simulink model "Copy_of_LQR_bloques_SS_LQR_cascada_PID_controller"  (R2023a)
settings: Solver=VariableStepAuto  StartTime=0.0  StopTime=2000  RelTol=1e-3
undefined symbols (not defined in the file): A, A_model, A_motor, B, B_mag0, B_model2, B_motor, C_model2, C_motor, D_motor, Gamma, I, J, K3_2, K4_2, K_gamma, Ke, Kt, La, n_cal, R_mgt, Ra, T_ext, T_max, T_max_mgt
libraries: slpidlib x7, matrix_library x5, simulink_extras x3, aerolibutil x1, vrlib x1
settings Model: Creator=Personal  LastModifiedBy=Personal
settings SolverCC: ZeroCrossAlgorithm=Adaptive
settings DebuggingCC: MaskedZcDiagnostic=none  IgnoredZcDiagnostic=none

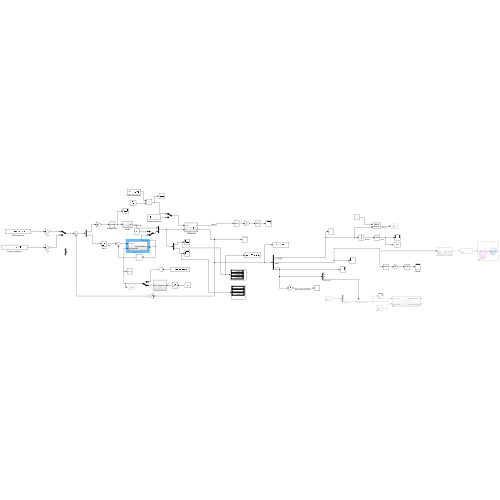
[thumbnail: Simulink's stored preview of the top-level diagram]
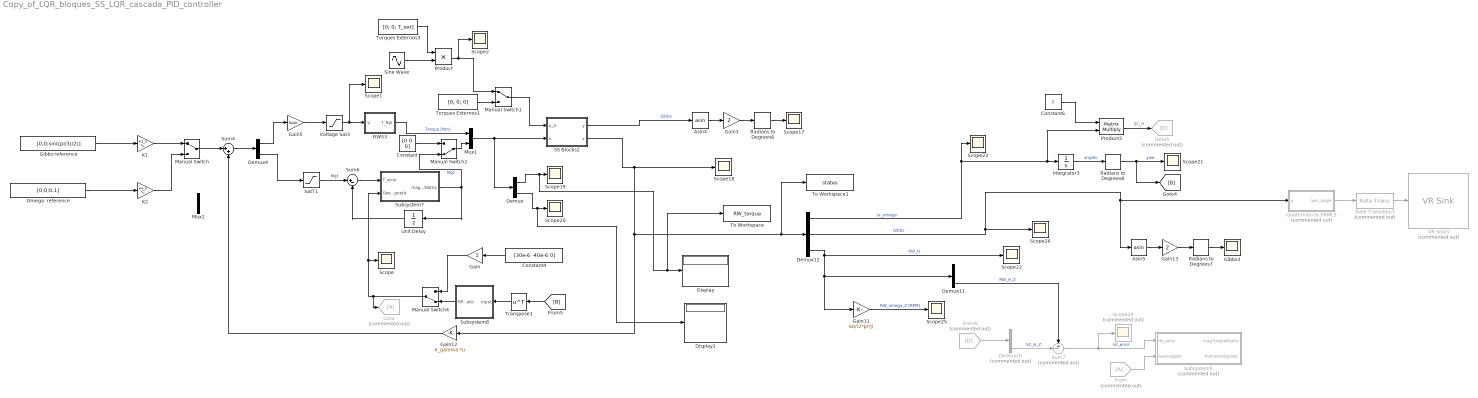
== system Copy_of_LQR_bloques_SS_LQR_cascada_PID_controller ==
  Asin4 : Trigonometry  Operator=asin
  Asin5 : Trigonometry  Operator=asin
  Constant : Constant  Value=[0 0 0]
  Constant4 : Constant  Value=[30e-6 -40e-6 0]
  Constant6 : Constant  Value=I
  Demux : Demux  Outputs=2
  Demux10 : Demux  Commented=on  Outputs=3
  Demux11 : Demux  Outputs=3
  Demux12 : Demux  Outputs=3
  Demux4 : Demux  Outputs=2
  Display : Display
  Display1 : Display
  From : From  Commented=on
  From6 : From  Commented=on  GotoTag=D
  Gain : Gain
  Gain11 : Gain  Gain=60/(2*pi*J)
  Gain12 : Gain  Gain=-K_gamma  Multiplication=Matrix(K*u)
  Gain13 : Gain  Gain=2
  Gain3 : Gain  Gain=2
  Gain5 : Gain  Gain=Ra/Kt
  Gibbs reference : Constant  Value=[0;0;sin((pi/3)/2)]
  Gibbs3 : Scope
  Goto : Goto  Commented=on
  Goto5 : Goto  Commented=on  GotoTag=D
  Integrator3 : Integrator  InitialCondition=[0 0 0]
  K1 : Gain  Gain=K3_2  Multiplication=Matrix(K*u)
  K2 : Gain  Gain=K4_2  Multiplication=Matrix(K*u)
  Manual Switch : ManualSwitch
  Manual Switch1 : ManualSwitch
  Manual Switch2 : ManualSwitch  CurrentSetting=0
  Manual Switch4 : ManualSwitch  CurrentSetting=0
  Mux1 : Mux  Inputs=2
  Mux2 : Mux  Inputs=2
  Omega  reference : Constant  Value=[0;0;0.1]
  Product : Product
  Product3 : Product  Multiplication=Matrix(*)
  Quaternion to VRML3 : Subsystem  Commented=on
  RWS3 : Subsystem
  Radians to Degrees6 : simulink_extras/Transformations/Radians to Degrees
  Radians to Degrees7 : simulink_extras/Transformations/Radians to Degrees
  Radians to Degrees8 : simulink_extras/Transformations/Radians to Degrees
  Rate Transition3 : RateTransition  Commented=on
  SS Blocks2 : Subsystem
  SatT1 : Saturate  UpperLimit=T_max_mgt  LowerLimit=-T_max_mgt
  Scope{,1..2,17..23,25..26} (12 alike) : Scope
  Scope24 : Scope  Commented=on
  Sine Wave : Sin  Frequency=0.05  SampleTime=0
  Subsystem7 : Subsystem
  Subsystem8 : Subsystem
  Subsystem9 : Subsystem  Commented=on
  Sum4 : Sum  Inputs=|++
  Sum6 : Sum  Inputs=|+-
  Sum7 : Sum  Commented=on  Inputs=+-|
  To Workspace : ToWorkspace  VariableName=RW_torque  SaveFormat=Structure With Time  SampleTime=-1
  To Workspace1 : ToWorkspace  VariableName=states  SaveFormat=Structure With Time  SampleTime=-1
  Torques Externos1 : Constant  Value=[0; 0; 0]
  Torques Externos3 : Constant  Value=[0; 0; T_ext]
  Transpose1 : Math  Operator=transpose
  Unit Delay : UnitDelay  SampleTime=-1  HasFrameUpgradeWarning=on
  VR Sink3 : vrlib/VR Sink  Commented=on  InstantiateOnLoad=on  SampleTime=0.1  ViewEnable=on  RemoteChange=off  RemoteView=off  FieldsWritten=STLB_Transform.rotation.4.1.1.double  WorldFileName=EscenarioCubeSat.x3d  AutoView=off  VideoDimensions=[]  AllowVariableSize=off  FigureProperties=[]
  Voltage Sat3 : Saturate  UpperLimit=6  LowerLimit=-6
  wires:
  Gibbs reference/1 -> K1/1
  K1/1 -> Manual Switch/1
  Mux1/1 -> Demux/1, SS Blocks2/2(u)
  Torques Externos3/1 -> Product/1
  Gain3/1 -> Radians to Degrees6/1
  SS Blocks2/1(y) -> Asin4/1  "Gibbs"
  Asin4/1 -> Gain3/1
  Radians to Degrees6/1 -> Scope17/1
  Demux/1 -> To Workspace/1, Display/1, Scope19/1
  Demux/2 -> Display1/1, Scope20/1
  Voltage Sat3/1 -> Scope1/1, RWS3/1(V)
  Gain5/1 -> Voltage Sat3/1
  SatT1/1 -> Sum6/1  "Mgt"
  Sum6/1 -> Subsystem7/1(T_error)
  Manual Switch4/1 -> Goto/1, Scope/1, Subsystem7/2(Geomagnetic)
  Demux4/1 -> Gain5/1
  Demux4/2 -> SatT1/1
  Gain12/1 -> Sum4/2
  Sum4/1 -> Demux4/1
  Subsystem7/1(magTorqueMatrix) -> Manual Switch2/2, Unit Delay/1  "Mgt"
  RWS3/1(T_RW) -> Mux1/1  "Torque [Nm]"
  Constant4/1 -> Gain/1
  Subsystem8/1(RPY_Magnetic) -> Manual Switch4/2
  Transpose1/1 -> Subsystem8/1(Input)
  Gain/1 -> Manual Switch4/1
  From6/1 -> Demux10/1
  SS Blocks2/2(x) -> Gain12/1, To Workspace1/1, Demux12/1, Scope18/1
  Radians to Degrees7/1 -> Gibbs3/1
  Demux10/3 -> Sum7/2  "SC_H_Z"
  Radians to Degrees8/1 -> [B], Scope21/1  "yaw"
  Demux11/3 -> Sum7/1  "RW_H_Z"
  Rate Transition3/1 -> VR Sink3/1
  Quaternion to VRML3/1(axis_angle) -> Rate Transition3/1
  Gain13/1 -> Radians to Degrees7/1
  Product3/1 -> Goto5/1  "SC_H"
  Integrator3/1 -> Radians to Degrees8/1  "angles"
  Gain11/1 -> Scope25/1  "RW_omega_Z [RPM]"
  Demux12/2 -> Asin5/1, Quaternion to VRML3/1(q), Scope26/1  "Gibbs"
  Sum7/1 -> Scope24/1, Subsystem9/1(Hz_error)  "Hz_error"
  Asin5/1 -> Gain13/1
  Constant6/1 -> Product3/1
  Demux12/3 -> Scope22/1, Gain11/1, Demux11/1  "RW_H"
  Demux12/1 -> Integrator3/1, Product3/2, Scope23/1  "sc_omega"
  [B] -> Transpose1/1
  Unit Delay/1 -> Sum6/2
  From/1 -> Subsystem9/2(Geomagetic)
  Omega  reference/1 -> K2/1
  Manual Switch/1 -> Sum4/1
  K2/1 -> Manual Switch/2
  Manual Switch1/1 -> SS Blocks2/1(u_d)
  Torques Externos1/1 -> Manual Switch1/2
  Constant/1 -> Manual Switch2/1
  Manual Switch2/1 -> Mux1/2
  Sine Wave/1 -> Product/2
  Product/1 -> Scope2/1, Manual Switch1/1

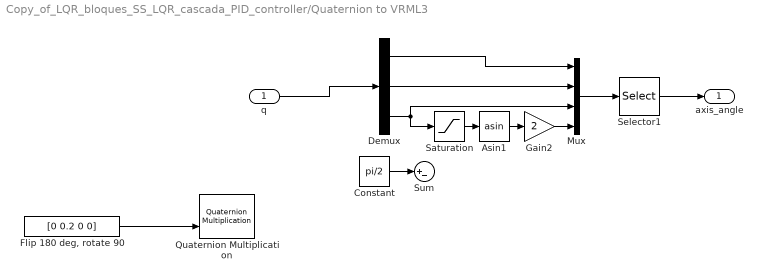
== system Copy_of_LQR_bloques_SS_LQR_cascada_PID_controller/Quaternion to VRML3 ==
  q : Inport
  Asin1 : Trigonometry  Operator=asin
  Constant : Constant  Value=pi/2
  Demux : Demux  Outputs=3
  "Flip 180 deg, rotate 90" : Constant  Value=[0 0.2 0 0]
  Gain2 : Gain  Gain=2
  Mux : Mux
  Quaternion Multiplication : aerolibutil/Quaternion Multiplication
  Saturation : Saturate
  Selector1 : Selector  InputPortWidth=4  IndexOptions=Index vector (dialog)  Indices=[2 3 1 4]  OutputSizes=1
  Sum : Sum  Inputs=|+-
  axis_angle : Outport  VectorParamsAs1DForOutWhenUnconnected=off
  wires:
  Constant/1 -> Sum/1
  Saturation/1 -> Asin1/1
  Asin1/1 -> Gain2/1
  Demux/3 -> Mux/3, Saturation/1
  Gain2/1 -> Mux/4
  Selector1/1 -> axis_angle/1
  Mux/1 -> Selector1/1
  Demux/1 -> Mux/1
  q/1 -> Demux/1
  "Flip 180 deg, rotate 90"/1 -> Quaternion Multiplication/2
  Demux/2 -> Mux/2

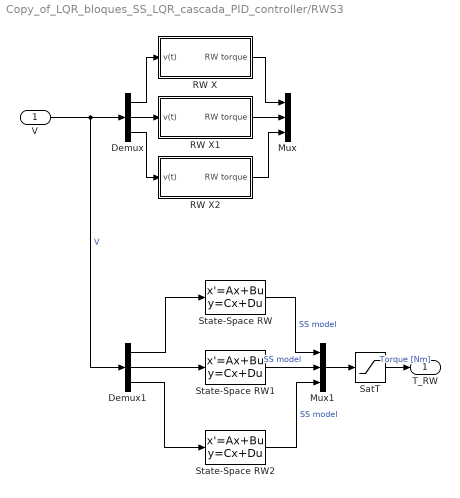
== system Copy_of_LQR_bloques_SS_LQR_cascada_PID_controller/RWS3 ==
  V : Inport
  Demux : Demux  Outputs=3
  Demux1 : Demux  Outputs=3
  Mux : Mux  Inputs=3
  Mux1 : Mux  Inputs=3
  RW X : Subsystem
  RW X1 : Subsystem
  RW X2 : Subsystem
  SatT : Saturate  UpperLimit=T_max  LowerLimit=-T_max
  State-Space RW : StateSpace  A=A_motor  B=B_motor  C=C_motor  D=D_motor  InitialCondition=0
  State-Space RW1 : StateSpace  A=A_motor  B=B_motor  C=C_motor  D=D_motor  InitialCondition=0
  State-Space RW2 : StateSpace  A=A_motor  B=B_motor  C=C_motor  D=D_motor  InitialCondition=0
  T_RW : Outport
  wires:
  Demux/1 -> RW X/1(v(t))
  V/1 -> Demux1/1, Demux/1  "V"
  Demux/3 -> RW X2/1(v(t))
  Demux/2 -> RW X1/1(v(t))
  RW X1/1(RW torque) -> Mux/2
  RW X2/1(RW torque) -> Mux/3
  RW X/1(RW torque) -> Mux/1
  Demux1/1 -> State-Space RW/1
  Demux1/2 -> State-Space RW1/1
  Demux1/3 -> State-Space RW2/1
  State-Space RW1/1 -> Mux1/2  "SS model"
  State-Space RW/1 -> Mux1/1  "SS model"
  State-Space RW2/1 -> Mux1/3  "SS model"
  Mux1/1 -> SatT/1
  SatT/1 -> T_RW/1  "Torque [Nm]"

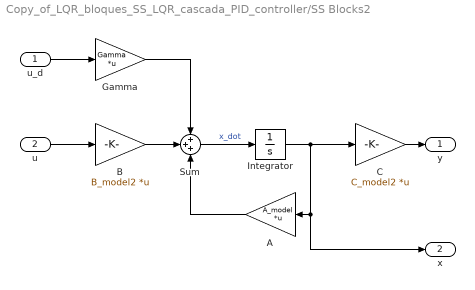
== system Copy_of_LQR_bloques_SS_LQR_cascada_PID_controller/SS Blocks2 ==
  u_d : Inport
  u : Inport  Port=2
  A : Gain  Gain=A_model  Multiplication=Matrix(K*u)
  B : Gain  Gain=B_model2  Multiplication=Matrix(K*u)
  C : Gain  Gain=C_model2  Multiplication=Matrix(K*u)
  Gamma : Gain  Gain=Gamma  Multiplication=Matrix(K*u)
  Integrator : Integrator  InitialCondition=zeros(9,1)
  Sum : Sum  Inputs=+++
  y : Outport
  x : Outport  Port=2
  wires:
  B/1 -> Sum/2
  u/1 -> B/1
  Sum/1 -> Integrator/1  "x_dot"
  A/1 -> Sum/3
  C/1 -> y/1
  Integrator/1 -> C/1, x/1, A/1
  u_d/1 -> Gamma/1
  Gamma/1 -> Sum/1

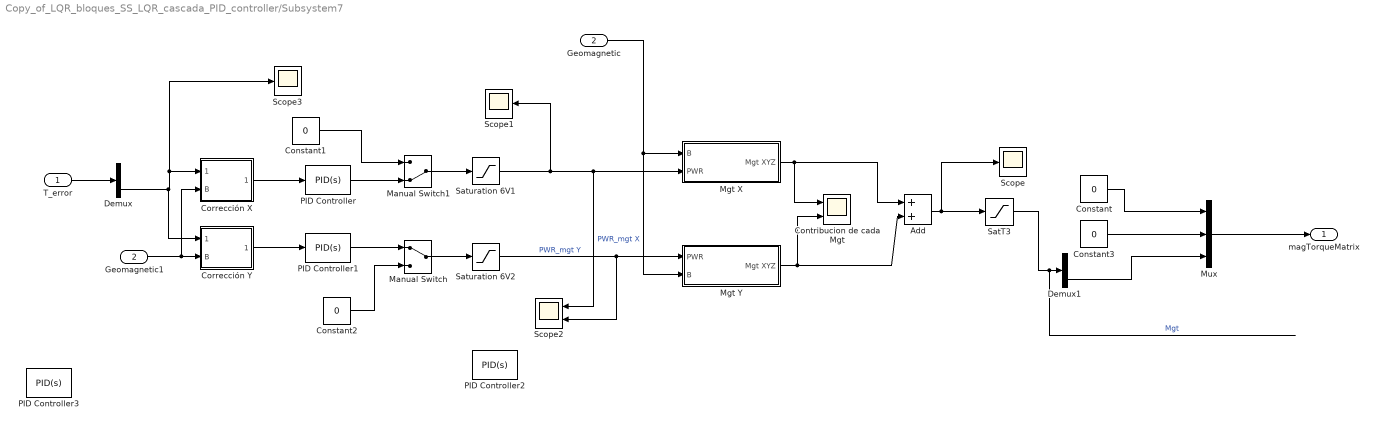
== system Copy_of_LQR_bloques_SS_LQR_cascada_PID_controller/Subsystem7 ==
  T_error : Inport
  Geomagnetic : Inport  Port=2
  Add : Sum
  Constant{,1..3} (4 alike) : Constant  Value=0
  Contribucion de cada Mgt : Scope  NumInputPorts=2
  Corrección X : MATLAB Function  TreatAsAtomicUnit=on
  Corrección Y : MATLAB Function  TreatAsAtomicUnit=on
  Demux : Demux  Outputs=3
  Demux1 : Demux  Outputs=3
  Geomagnetic1 : InportShadow  Port=2
  Manual Switch : ManualSwitch
  Manual Switch1 : ManualSwitch  CurrentSetting=0
  Mgt X : Subsystem
  Mgt Y : Subsystem
  Mux : Mux  Inputs=3
  PID Controller : slpidlib/PID Controller  Controller=PID  Form=Parallel  TimeDomain=Continuous-time  UseExternalTs=off  SampleTime=-1  IntegratorMethod=Forward Euler  FilterMethod=Forward Euler  ControllerParametersSource=internal  P=45000  I=500000  UseKiTs=off  D=8000  N=100  UseFilter=on  TunerSelectOption=Transfer Function Based (PID Tuner App)  InitialConditionSource=internal  InitialConditionForIntegrator=0  InitialConditionForFilter=0  DifferentiatorICPrevScaledInput=0  ExternalReset=none  TrackingMode=off  Kt=1  LimitOutput=on  SatLimitsSource=internal  UpperSaturationLimit=5  LowerSaturationLimit=-5  LinearizeAsGain=on  AntiWindupMode=none  Kb=1  LimitIntegrator=off  UpperIntegratorSaturationLimit=inf  LowerIntegratorSaturationLimit=-inf  POutMin=[]  POutMax=[]  IOutMin=[]  IOutMax=[]  DOutMin=[]  DOutMax=[]  NOutMin=[]  NOutMax=[]  SumOutMin=[]  SumOutMax=[]  SaturationOutMin=[]  SaturationOutMax=[]  PParamMin=[]  PParamMax=[]  IParamMin=[]  IParamMax=[]  DParamMin=[]  DParamMax=[]  NParamMin=[]  NParamMax=[]  KbParamMin=[]  KbParamMax=[]  KtParamMin=[]  KtParamMax=[]  KbOutMin=[]  KbOutMax=[]  KtOutMin=[]  KtOutMax=[]  IntegratorOutMin=[]  IntegratorOutMax=[]  FilterOutMin=[]  FilterOutMax=[]  SumI1OutMin=[]  SumI1OutMax=[]  SumI2OutMin=[]  SumI2OutMax=[]  SumI3OutMin=[]  SumI3OutMax=[]  SumI4OutMin=[]  SumI4OutMax=[]  SumDOutMin=[]  SumDOutMax=[]  DifferentiatorOutMin=[]  DifferentiatorOutMax=[]  FilterDiffOutCoefMin=[]  FilterDiffOutCoefMax=[]  ReciprocalOutMin=[]  ReciprocalOutMax=[]  SumDenOutMin=[]  SumDenOutMax=[]  SumNumOutMin=[]  SumNumOutMax=[]  DivideOutMin=[]  DivideOutMax=[]  UdiffTsProdOutMin=[]  UdiffTsProdOutMax=[]  NTsProdOutMin=[]  NTsProdOutMax=[]  UintegralTsProdOutMin=[]  UintegralTsProdOutMax=[]  UngainTsProdOutMin=[]  UngainTsProdOutMax=[]  ClampingZeroOutDataTypeStr=Inherit: Inherit via back propagation  ClampingZeroOutMin=[]  ClampingZeroOutMax=[]  FilterDenConstantOutDataTypeStr=Inherit: Inherit via back propagation  FilterDenConstantOutMin=[]  FilterDenConstantOutMax=[]  PCopyOutDataTypeStr=Inherit: Inherit via back propagation  PCopyOutMin=[]  PCopyOutMax=[]  NCopyOutDataTypeStr=Inherit: Inherit via back propagation  NCopyOutMin=[]  NCopyOutMax=[]  IntegratorContinuousStateAttributes=''  IntegratorStateMustResolveToSignalObject=off  IntegratorRTWStateStorageClass=Auto  FilterContinuousStateAttributes=''  FilterStateMustResolveToSignalObject=off  FilterRTWStateStorageClass=Auto  ParallelPVariant=InternalParameters  IdealPVariant=Disabled  IVariant=InternalParameters  DVariant=InternalParameters  IntegratorVariant=Continuous  SatVariant=Enabled  AWVariant=Passthrough  PCopyVariant=Disabled  TRVariant=Disabled  FdbkBlocksVariant=Forward  IdealPFdbkVariant=Disabled  SatFdbkVariant=Disabled  DerivativeFilterVariant=ContFilter  NVariant=InternalParameters  NCopyVariant=Disabled  FilterICVariant=InternalICsFilter  IntegratorICVariant=InternalICs  ExternalResetVariant=Disabled  TRSumVariant=Passthrough  SumFdbkVariant=Disabled  SumVariant=Sum_PID  TsampFilterVariant=InternalTs  TsampNgainVariant=Passthrough  TsampIntegralVariant=Disabled_SignalSpec  ExternalSaturationOutDataTypeStr=Inherit: Same as second input
  PID Controller1 : slpidlib/PID Controller  Controller=PID  Form=Parallel  TimeDomain=Continuous-time  UseExternalTs=off  SampleTime=-1  IntegratorMethod=Forward Euler  FilterMethod=Forward Euler  ControllerParametersSource=internal  P=45000  I=500000  UseKiTs=off  D=8000  N=100  UseFilter=on  TunerSelectOption=Transfer Function Based (PID Tuner App)  InitialConditionSource=internal  InitialConditionForIntegrator=0  InitialConditionForFilter=0  DifferentiatorICPrevScaledInput=0  ExternalReset=none  TrackingMode=off  Kt=1  LimitOutput=on  SatLimitsSource=internal  UpperSaturationLimit=5  LowerSaturationLimit=-5  LinearizeAsGain=on  AntiWindupMode=none  Kb=1  LimitIntegrator=off  UpperIntegratorSaturationLimit=inf  LowerIntegratorSaturationLimit=-inf  POutMin=[]  POutMax=[]  IOutMin=[]  IOutMax=[]  DOutMin=[]  DOutMax=[]  NOutMin=[]  NOutMax=[]  SumOutMin=[]  SumOutMax=[]  SaturationOutMin=[]  SaturationOutMax=[]  PParamMin=[]  PParamMax=[]  IParamMin=[]  IParamMax=[]  DParamMin=[]  DParamMax=[]  NParamMin=[]  NParamMax=[]  KbParamMin=[]  KbParamMax=[]  KtParamMin=[]  KtParamMax=[]  KbOutMin=[]  KbOutMax=[]  KtOutMin=[]  KtOutMax=[]  IntegratorOutMin=[]  IntegratorOutMax=[]  FilterOutMin=[]  FilterOutMax=[]  SumI1OutMin=[]  SumI1OutMax=[]  SumI2OutMin=[]  SumI2OutMax=[]  SumI3OutMin=[]  SumI3OutMax=[]  SumI4OutMin=[]  SumI4OutMax=[]  SumDOutMin=[]  SumDOutMax=[]  DifferentiatorOutMin=[]  DifferentiatorOutMax=[]  FilterDiffOutCoefMin=[]  FilterDiffOutCoefMax=[]  ReciprocalOutMin=[]  ReciprocalOutMax=[]  SumDenOutMin=[]  SumDenOutMax=[]  SumNumOutMin=[]  SumNumOutMax=[]  DivideOutMin=[]  DivideOutMax=[]  UdiffTsProdOutMin=[]  UdiffTsProdOutMax=[]  NTsProdOutMin=[]  NTsProdOutMax=[]  UintegralTsProdOutMin=[]  UintegralTsProdOutMax=[]  UngainTsProdOutMin=[]  UngainTsProdOutMax=[]  ClampingZeroOutDataTypeStr=Inherit: Inherit via back propagation  ClampingZeroOutMin=[]  ClampingZeroOutMax=[]  FilterDenConstantOutDataTypeStr=Inherit: Inherit via back propagation  FilterDenConstantOutMin=[]  FilterDenConstantOutMax=[]  PCopyOutDataTypeStr=Inherit: Inherit via back propagation  PCopyOutMin=[]  PCopyOutMax=[]  NCopyOutDataTypeStr=Inherit: Inherit via back propagation  NCopyOutMin=[]  NCopyOutMax=[]  IntegratorContinuousStateAttributes=''  IntegratorStateMustResolveToSignalObject=off  IntegratorRTWStateStorageClass=Auto  FilterContinuousStateAttributes=''  FilterStateMustResolveToSignalObject=off  FilterRTWStateStorageClass=Auto  ParallelPVariant=InternalParameters  IdealPVariant=Disabled  IVariant=InternalParameters  DVariant=InternalParameters  IntegratorVariant=Continuous  SatVariant=Enabled  AWVariant=Passthrough  PCopyVariant=Disabled  TRVariant=Disabled  FdbkBlocksVariant=Forward  IdealPFdbkVariant=Disabled  SatFdbkVariant=Disabled  DerivativeFilterVariant=ContFilter  NVariant=InternalParameters  NCopyVariant=Disabled  FilterICVariant=InternalICsFilter  IntegratorICVariant=InternalICs  ExternalResetVariant=Disabled  TRSumVariant=Passthrough  SumFdbkVariant=Disabled  SumVariant=Sum_PID  TsampFilterVariant=InternalTs  TsampNgainVariant=Passthrough  TsampIntegralVariant=Disabled_SignalSpec  ExternalSaturationOutDataTypeStr=Inherit: Same as second input
  PID Controller2 : slpidlib/PID Controller  Controller=PID  Form=Parallel  TimeDomain=Continuous-time  UseExternalTs=off  SampleTime=-1  IntegratorMethod=Forward Euler  FilterMethod=Forward Euler  ControllerParametersSource=internal  P=0  I=2538362.26384975  UseKiTs=off  D=0  N=100  UseFilter=on  TunerSelectOption=Transfer Function Based (PID Tuner App)  InitialConditionSource=internal  InitialConditionForIntegrator=0  InitialConditionForFilter=0  DifferentiatorICPrevScaledInput=0  ExternalReset=none  TrackingMode=off  Kt=1  LimitOutput=on  SatLimitsSource=internal  UpperSaturationLimit=5  LowerSaturationLimit=-5  LinearizeAsGain=on  AntiWindupMode=clamping  Kb=1  LimitIntegrator=off  UpperIntegratorSaturationLimit=inf  LowerIntegratorSaturationLimit=-inf  POutMin=[]  POutMax=[]  IOutMin=[]  IOutMax=[]  DOutMin=[]  DOutMax=[]  NOutMin=[]  NOutMax=[]  SumOutMin=[]  SumOutMax=[]  SaturationOutMin=[]  SaturationOutMax=[]  PParamMin=[]  PParamMax=[]  IParamMin=[]  IParamMax=[]  DParamMin=[]  DParamMax=[]  NParamMin=[]  NParamMax=[]  KbParamMin=[]  KbParamMax=[]  KtParamMin=[]  KtParamMax=[]  KbOutMin=[]  KbOutMax=[]  KtOutMin=[]  KtOutMax=[]  IntegratorOutMin=[]  IntegratorOutMax=[]  FilterOutMin=[]  FilterOutMax=[]  SumI1OutMin=[]  SumI1OutMax=[]  SumI2OutMin=[]  SumI2OutMax=[]  SumI3OutMin=[]  SumI3OutMax=[]  SumI4OutMin=[]  SumI4OutMax=[]  SumDOutMin=[]  SumDOutMax=[]  DifferentiatorOutMin=[]  DifferentiatorOutMax=[]  FilterDiffOutCoefMin=[]  FilterDiffOutCoefMax=[]  ReciprocalOutMin=[]  ReciprocalOutMax=[]  SumDenOutMin=[]  SumDenOutMax=[]  SumNumOutMin=[]  SumNumOutMax=[]  DivideOutMin=[]  DivideOutMax=[]  UdiffTsProdOutMin=[]  UdiffTsProdOutMax=[]  NTsProdOutMin=[]  NTsProdOutMax=[]  UintegralTsProdOutMin=[]  UintegralTsProdOutMax=[]  UngainTsProdOutMin=[]  UngainTsProdOutMax=[]  ClampingZeroOutDataTypeStr=Inherit: Inherit via back propagation  ClampingZeroOutMin=[]  ClampingZeroOutMax=[]  FilterDenConstantOutDataTypeStr=Inherit: Inherit via back propagation  FilterDenConstantOutMin=[]  FilterDenConstantOutMax=[]  PCopyOutDataTypeStr=Inherit: Inherit via back propagation  PCopyOutMin=[]  PCopyOutMax=[]  NCopyOutDataTypeStr=Inherit: Inherit via back propagation  NCopyOutMin=[]  NCopyOutMax=[]  IntegratorContinuousStateAttributes=''  IntegratorStateMustResolveToSignalObject=off  IntegratorRTWStateStorageClass=Auto  FilterContinuousStateAttributes=''  FilterStateMustResolveToSignalObject=off  FilterRTWStateStorageClass=Auto  ParallelPVariant=InternalParameters  IdealPVariant=Disabled  IVariant=InternalParameters  DVariant=InternalParameters  IntegratorVariant=Continuous  SatVariant=Enabled  AWVariant=ContClampingParallel  PCopyVariant=Disabled  TRVariant=Disabled  FdbkBlocksVariant=Forward  IdealPFdbkVariant=Disabled  SatFdbkVariant=Disabled  DerivativeFilterVariant=ContFilter  NVariant=InternalParameters  NCopyVariant=Disabled  FilterICVariant=InternalICsFilter  IntegratorICVariant=InternalICs  ExternalResetVariant=Disabled  TRSumVariant=Passthrough  SumFdbkVariant=Disabled  SumVariant=Sum_PID  TsampFilterVariant=InternalTs  TsampNgainVariant=Passthrough  TsampIntegralVariant=Disabled_SignalSpec  ExternalSaturationOutDataTypeStr=Inherit: Same as second input
  PID Controller3 : slpidlib/PID Controller  Controller=PID  Form=Parallel  TimeDomain=Continuous-time  UseExternalTs=off  SampleTime=-1  IntegratorMethod=Forward Euler  FilterMethod=Forward Euler  ControllerParametersSource=internal  P=500000  I=30000  UseKiTs=off  D=2500  N=100  UseFilter=on  TunerSelectOption=Transfer Function Based (PID Tuner App)  InitialConditionSource=internal  InitialConditionForIntegrator=0  InitialConditionForFilter=0  DifferentiatorICPrevScaledInput=0  ExternalReset=none  TrackingMode=off  Kt=1  LimitOutput=off  SatLimitsSource=internal  UpperSaturationLimit=1  LowerSaturationLimit=-1  LinearizeAsGain=on  AntiWindupMode=none  Kb=1  LimitIntegrator=off  UpperIntegratorSaturationLimit=inf  LowerIntegratorSaturationLimit=-inf  POutMin=[]  POutMax=[]  IOutMin=[]  IOutMax=[]  DOutMin=[]  DOutMax=[]  NOutMin=[]  NOutMax=[]  SumOutMin=[]  SumOutMax=[]  SaturationOutMin=[]  SaturationOutMax=[]  PParamMin=[]  PParamMax=[]  IParamMin=[]  IParamMax=[]  DParamMin=[]  DParamMax=[]  NParamMin=[]  NParamMax=[]  KbParamMin=[]  KbParamMax=[]  KtParamMin=[]  KtParamMax=[]  KbOutMin=[]  KbOutMax=[]  KtOutMin=[]  KtOutMax=[]  IntegratorOutMin=[]  IntegratorOutMax=[]  FilterOutMin=[]  FilterOutMax=[]  SumI1OutMin=[]  SumI1OutMax=[]  SumI2OutMin=[]  SumI2OutMax=[]  SumI3OutMin=[]  SumI3OutMax=[]  SumI4OutMin=[]  SumI4OutMax=[]  SumDOutMin=[]  SumDOutMax=[]  DifferentiatorOutMin=[]  DifferentiatorOutMax=[]  FilterDiffOutCoefMin=[]  FilterDiffOutCoefMax=[]  ReciprocalOutMin=[]  ReciprocalOutMax=[]  SumDenOutMin=[]  SumDenOutMax=[]  SumNumOutMin=[]  SumNumOutMax=[]  DivideOutMin=[]  DivideOutMax=[]  UdiffTsProdOutMin=[]  UdiffTsProdOutMax=[]  NTsProdOutMin=[]  NTsProdOutMax=[]  UintegralTsProdOutMin=[]  UintegralTsProdOutMax=[]  UngainTsProdOutMin=[]  UngainTsProdOutMax=[]  ClampingZeroOutDataTypeStr=Inherit: Inherit via back propagation  ClampingZeroOutMin=[]  ClampingZeroOutMax=[]  FilterDenConstantOutDataTypeStr=Inherit: Inherit via back propagation  FilterDenConstantOutMin=[]  FilterDenConstantOutMax=[]  PCopyOutDataTypeStr=Inherit: Inherit via back propagation  PCopyOutMin=[]  PCopyOutMax=[]  NCopyOutDataTypeStr=Inherit: Inherit via back propagation  NCopyOutMin=[]  NCopyOutMax=[]  IntegratorContinuousStateAttributes=''  IntegratorStateMustResolveToSignalObject=off  IntegratorRTWStateStorageClass=Auto  FilterContinuousStateAttributes=''  FilterStateMustResolveToSignalObject=off  FilterRTWStateStorageClass=Auto  ParallelPVariant=InternalParameters  IdealPVariant=Disabled  IVariant=InternalParameters  DVariant=InternalParameters  IntegratorVariant=Continuous  SatVariant=Disabled  AWVariant=Passthrough  PCopyVariant=Disabled  TRVariant=Disabled  FdbkBlocksVariant=Forward  IdealPFdbkVariant=Disabled  SatFdbkVariant=Disabled  DerivativeFilterVariant=ContFilter  NVariant=InternalParameters  NCopyVariant=Disabled  FilterICVariant=InternalICsFilter  IntegratorICVariant=InternalICs  ExternalResetVariant=Disabled  TRSumVariant=Passthrough  SumFdbkVariant=Disabled  SumVariant=Sum_PID  TsampFilterVariant=InternalTs  TsampNgainVariant=Passthrough  TsampIntegralVariant=Disabled_SignalSpec  ExternalSaturationOutDataTypeStr=Inherit: Same as second input
  SatT3 : Saturate  UpperLimit=T_max_mgt  LowerLimit=-T_max_mgt
  Saturation 6V1 : Saturate  UpperLimit=5  LowerLimit=-5
  Saturation 6V2 : Saturate  UpperLimit=5  LowerLimit=-5
  Scope : Scope
  Scope1 : Scope
  Scope2 : Scope  NumInputPorts=2
  Scope3 : Scope
  magTorqueMatrix : Outport
  wires:
  PID Controller/1 -> Manual Switch1/2
  Saturation 6V1/1 -> Scope2/1, Mgt X/2(PWR), Scope1/1  "PWR_mgt X"
  Geomagnetic/1 -> Mgt Y/2(B), Mgt X/1(B)
  Manual Switch/1 -> Saturation 6V2/1
  Constant1/1 -> Manual Switch1/1
  Manual Switch1/1 -> Saturation 6V1/1
  Saturation 6V2/1 -> Scope2/2, Mgt Y/1(PWR)  "PWR_mgt Y"
  Add/1 -> SatT3/1, Scope/1
  T_error/1 -> Demux/1
  Mgt X/1(Mgt XYZ) -> Contribucion de cada Mgt/1, Add/1
  Mgt Y/1(Mgt XYZ) -> Add/2, Contribucion de cada Mgt/2
  Constant2/1 -> Manual Switch/2
  Demux/3 -> Corrección Y/1("T_error "), Corrección X/1("T_error "), Scope3/1
  SatT3/1 -> Demux1/1  "Mgt"
  Corrección X/1(T_error) -> PID Controller/1
  Geomagnetic1/1 -> Corrección X/2(B), Corrección Y/2(B)
  Demux1/3 -> Mux/3
  Constant/1 -> Mux/1
  Constant3/1 -> Mux/2
  Mux/1 -> magTorqueMatrix/1
  Corrección Y/1(T_error) -> PID Controller1/1
  PID Controller1/1 -> Manual Switch/1

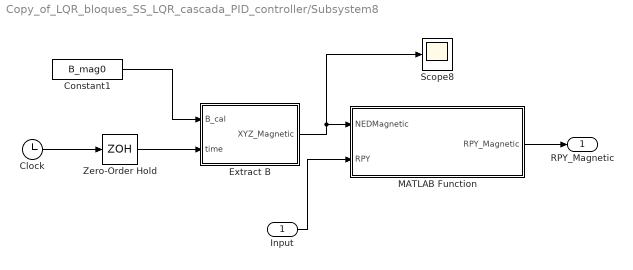
== system Copy_of_LQR_bloques_SS_LQR_cascada_PID_controller/Subsystem8 ==
  Input : Inport
  Clock : Clock
  Constant1 : Constant  Value=B_mag0
  Extract B : MATLAB Function  TreatAsAtomicUnit=on
  MATLAB Function : MATLAB Function  TreatAsAtomicUnit=on
  Scope8 : Scope
  Zero-Order Hold : ZeroOrderHold  SampleTime=-1
  RPY_Magnetic : Outport
  wires:
  Constant1/1 -> Extract B/1(B_cal)
  Extract B/1(XYZ_Magnetic) -> MATLAB Function/1(NEDMagnetic), Scope8/1
  Input/1 -> MATLAB Function/2(RPY)
  Zero-Order Hold/1 -> Extract B/2(time)
  MATLAB Function/1(RPY_Magnetic) -> RPY_Magnetic/1
  Clock/1 -> Zero-Order Hold/1

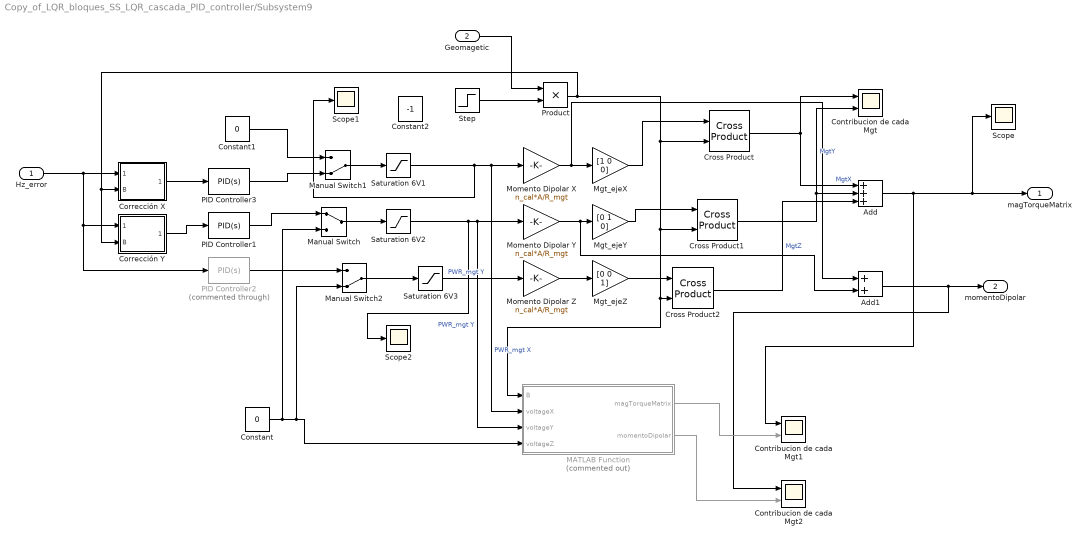
== system Copy_of_LQR_bloques_SS_LQR_cascada_PID_controller/Subsystem9 ==
  Hz_error : Inport
  Geomagetic : Inport  Port=2
  Add : Sum  Inputs=+++
  Add1 : Sum
  Constant : Constant  Value=0
  Constant1 : Constant  Value=0
  Constant2 : Constant  Value=-1
  Contribucion de cada Mgt : Scope  NumInputPorts=2
  Contribucion de cada Mgt1 : Scope  NumInputPorts=2
  Contribucion de cada Mgt2 : Scope  NumInputPorts=2
  Corrección X : MATLAB Function  TreatAsAtomicUnit=on
  Corrección Y : MATLAB Function  TreatAsAtomicUnit=on
  Cross Product : matrix_library/Cross Product
  Cross Product1 : matrix_library/Cross Product
  Cross Product2 : matrix_library/Cross Product
  MATLAB Function : MATLAB Function  Commented=on  TreatAsAtomicUnit=on
  Manual Switch : ManualSwitch
  Manual Switch1 : ManualSwitch  CurrentSetting=0
  Manual Switch2 : ManualSwitch  CurrentSetting=0
  Mgt_ejeX : Gain  Gain=[1 0 0]
  Mgt_ejeY : Gain  Gain=[0 1 0]
  Mgt_ejeZ : Gain  Gain=[0 0 1]
  Momento Dipolar X : Gain  Gain=n_cal*A/R_mgt
  Momento Dipolar Y : Gain  Gain=n_cal*A/R_mgt
  Momento Dipolar Z : Gain  Gain=n_cal*A/R_mgt
  PID Controller1 : slpidlib/PID Controller  Controller=PID  Form=Parallel  TimeDomain=Continuous-time  UseExternalTs=off  SampleTime=-1  IntegratorMethod=Forward Euler  FilterMethod=Forward Euler  ControllerParametersSource=internal  P=4500  I=800  UseKiTs=off  D=8000  N=100  UseFilter=on  TunerSelectOption=Transfer Function Based (PID Tuner App)  InitialConditionSource=internal  InitialConditionForIntegrator=0  InitialConditionForFilter=0  DifferentiatorICPrevScaledInput=0  ExternalReset=none  TrackingMode=off  Kt=1  LimitOutput=off  SatLimitsSource=internal  UpperSaturationLimit=1  LowerSaturationLimit=-1  LinearizeAsGain=on  AntiWindupMode=none  Kb=1  LimitIntegrator=off  UpperIntegratorSaturationLimit=inf  LowerIntegratorSaturationLimit=-inf  POutMin=[]  POutMax=[]  IOutMin=[]  IOutMax=[]  DOutMin=[]  DOutMax=[]  NOutMin=[]  NOutMax=[]  SumOutMin=[]  SumOutMax=[]  SaturationOutMin=[]  SaturationOutMax=[]  PParamMin=[]  PParamMax=[]  IParamMin=[]  IParamMax=[]  DParamMin=[]  DParamMax=[]  NParamMin=[]  NParamMax=[]  KbParamMin=[]  KbParamMax=[]  KtParamMin=[]  KtParamMax=[]  KbOutMin=[]  KbOutMax=[]  KtOutMin=[]  KtOutMax=[]  IntegratorOutMin=[]  IntegratorOutMax=[]  FilterOutMin=[]  FilterOutMax=[]  SumI1OutMin=[]  SumI1OutMax=[]  SumI2OutMin=[]  SumI2OutMax=[]  SumI3OutMin=[]  SumI3OutMax=[]  SumI4OutMin=[]  SumI4OutMax=[]  SumDOutMin=[]  SumDOutMax=[]  DifferentiatorOutMin=[]  DifferentiatorOutMax=[]  FilterDiffOutCoefMin=[]  FilterDiffOutCoefMax=[]  ReciprocalOutMin=[]  ReciprocalOutMax=[]  SumDenOutMin=[]  SumDenOutMax=[]  SumNumOutMin=[]  SumNumOutMax=[]  DivideOutMin=[]  DivideOutMax=[]  UdiffTsProdOutMin=[]  UdiffTsProdOutMax=[]  NTsProdOutMin=[]  NTsProdOutMax=[]  UintegralTsProdOutMin=[]  UintegralTsProdOutMax=[]  UngainTsProdOutMin=[]  UngainTsProdOutMax=[]  ClampingZeroOutDataTypeStr=Inherit: Inherit via back propagation  ClampingZeroOutMin=[]  ClampingZeroOutMax=[]  FilterDenConstantOutDataTypeStr=Inherit: Inherit via back propagation  FilterDenConstantOutMin=[]  FilterDenConstantOutMax=[]  PCopyOutDataTypeStr=Inherit: Inherit via back propagation  PCopyOutMin=[]  PCopyOutMax=[]  NCopyOutDataTypeStr=Inherit: Inherit via back propagation  NCopyOutMin=[]  NCopyOutMax=[]  IntegratorContinuousStateAttributes=''  IntegratorStateMustResolveToSignalObject=off  IntegratorRTWStateStorageClass=Auto  FilterContinuousStateAttributes=''  FilterStateMustResolveToSignalObject=off  FilterRTWStateStorageClass=Auto  ParallelPVariant=InternalParameters  IdealPVariant=Disabled  IVariant=InternalParameters  DVariant=InternalParameters  IntegratorVariant=Continuous  SatVariant=Disabled  AWVariant=Passthrough  PCopyVariant=Disabled  TRVariant=Disabled  FdbkBlocksVariant=Forward  IdealPFdbkVariant=Disabled  SatFdbkVariant=Disabled  DerivativeFilterVariant=ContFilter  NVariant=InternalParameters  NCopyVariant=Disabled  FilterICVariant=InternalICsFilter  IntegratorICVariant=InternalICs  ExternalResetVariant=Disabled  TRSumVariant=Passthrough  SumFdbkVariant=Disabled  SumVariant=Sum_PID  TsampFilterVariant=InternalTs  TsampNgainVariant=Passthrough  TsampIntegralVariant=Disabled_SignalSpec  ExternalSaturationOutDataTypeStr=Inherit: Same as second input
  PID Controller2 : slpidlib/PID Controller  Commented=through  Controller=PID  Form=Parallel  TimeDomain=Continuous-time  UseExternalTs=off  SampleTime=-1  IntegratorMethod=Forward Euler  FilterMethod=Forward Euler  ControllerParametersSource=internal  P=4500  I=800  UseKiTs=off  D=8000  N=100  UseFilter=on  TunerSelectOption=Transfer Function Based (PID Tuner App)  InitialConditionSource=internal  InitialConditionForIntegrator=0  InitialConditionForFilter=0  DifferentiatorICPrevScaledInput=0  ExternalReset=none  TrackingMode=off  Kt=1  LimitOutput=off  SatLimitsSource=internal  UpperSaturationLimit=1  LowerSaturationLimit=-1  LinearizeAsGain=on  AntiWindupMode=none  Kb=1  LimitIntegrator=off  UpperIntegratorSaturationLimit=inf  LowerIntegratorSaturationLimit=-inf  POutMin=[]  POutMax=[]  IOutMin=[]  IOutMax=[]  DOutMin=[]  DOutMax=[]  NOutMin=[]  NOutMax=[]  SumOutMin=[]  SumOutMax=[]  SaturationOutMin=[]  SaturationOutMax=[]  PParamMin=[]  PParamMax=[]  IParamMin=[]  IParamMax=[]  DParamMin=[]  DParamMax=[]  NParamMin=[]  NParamMax=[]  KbParamMin=[]  KbParamMax=[]  KtParamMin=[]  KtParamMax=[]  KbOutMin=[]  KbOutMax=[]  KtOutMin=[]  KtOutMax=[]  IntegratorOutMin=[]  IntegratorOutMax=[]  FilterOutMin=[]  FilterOutMax=[]  SumI1OutMin=[]  SumI1OutMax=[]  SumI2OutMin=[]  SumI2OutMax=[]  SumI3OutMin=[]  SumI3OutMax=[]  SumI4OutMin=[]  SumI4OutMax=[]  SumDOutMin=[]  SumDOutMax=[]  DifferentiatorOutMin=[]  DifferentiatorOutMax=[]  FilterDiffOutCoefMin=[]  FilterDiffOutCoefMax=[]  ReciprocalOutMin=[]  ReciprocalOutMax=[]  SumDenOutMin=[]  SumDenOutMax=[]  SumNumOutMin=[]  SumNumOutMax=[]  DivideOutMin=[]  DivideOutMax=[]  UdiffTsProdOutMin=[]  UdiffTsProdOutMax=[]  NTsProdOutMin=[]  NTsProdOutMax=[]  UintegralTsProdOutMin=[]  UintegralTsProdOutMax=[]  UngainTsProdOutMin=[]  UngainTsProdOutMax=[]  ClampingZeroOutDataTypeStr=Inherit: Inherit via back propagation  ClampingZeroOutMin=[]  ClampingZeroOutMax=[]  FilterDenConstantOutDataTypeStr=Inherit: Inherit via back propagation  FilterDenConstantOutMin=[]  FilterDenConstantOutMax=[]  PCopyOutDataTypeStr=Inherit: Inherit via back propagation  PCopyOutMin=[]  PCopyOutMax=[]  NCopyOutDataTypeStr=Inherit: Inherit via back propagation  NCopyOutMin=[]  NCopyOutMax=[]  IntegratorContinuousStateAttributes=''  IntegratorStateMustResolveToSignalObject=off  IntegratorRTWStateStorageClass=Auto  FilterContinuousStateAttributes=''  FilterStateMustResolveToSignalObject=off  FilterRTWStateStorageClass=Auto  ParallelPVariant=InternalParameters  IdealPVariant=Disabled  IVariant=InternalParameters  DVariant=InternalParameters  IntegratorVariant=Continuous  SatVariant=Disabled  AWVariant=Passthrough  PCopyVariant=Disabled  TRVariant=Disabled  FdbkBlocksVariant=Forward  IdealPFdbkVariant=Disabled  SatFdbkVariant=Disabled  DerivativeFilterVariant=ContFilter  NVariant=InternalParameters  NCopyVariant=Disabled  FilterICVariant=InternalICsFilter  IntegratorICVariant=InternalICs  ExternalResetVariant=Disabled  TRSumVariant=Passthrough  SumFdbkVariant=Disabled  SumVariant=Sum_PID  TsampFilterVariant=InternalTs  TsampNgainVariant=Passthrough  TsampIntegralVariant=Disabled_SignalSpec  ExternalSaturationOutDataTypeStr=Inherit: Same as second input
  PID Controller3 : slpidlib/PID Controller  Controller=PID  Form=Parallel  TimeDomain=Continuous-time  UseExternalTs=off  SampleTime=-1  IntegratorMethod=Forward Euler  FilterMethod=Forward Euler  ControllerParametersSource=internal  P=4500  I=800  UseKiTs=off  D=8000  N=100  UseFilter=on  TunerSelectOption=Transfer Function Based (PID Tuner App)  InitialConditionSource=internal  InitialConditionForIntegrator=0  InitialConditionForFilter=0  DifferentiatorICPrevScaledInput=0  ExternalReset=none  TrackingMode=off  Kt=1  LimitOutput=off  SatLimitsSource=internal  UpperSaturationLimit=1  LowerSaturationLimit=-1  LinearizeAsGain=on  AntiWindupMode=none  Kb=1  LimitIntegrator=off  UpperIntegratorSaturationLimit=inf  LowerIntegratorSaturationLimit=-inf  POutMin=[]  POutMax=[]  IOutMin=[]  IOutMax=[]  DOutMin=[]  DOutMax=[]  NOutMin=[]  NOutMax=[]  SumOutMin=[]  SumOutMax=[]  SaturationOutMin=[]  SaturationOutMax=[]  PParamMin=[]  PParamMax=[]  IParamMin=[]  IParamMax=[]  DParamMin=[]  DParamMax=[]  NParamMin=[]  NParamMax=[]  KbParamMin=[]  KbParamMax=[]  KtParamMin=[]  KtParamMax=[]  KbOutMin=[]  KbOutMax=[]  KtOutMin=[]  KtOutMax=[]  IntegratorOutMin=[]  IntegratorOutMax=[]  FilterOutMin=[]  FilterOutMax=[]  SumI1OutMin=[]  SumI1OutMax=[]  SumI2OutMin=[]  SumI2OutMax=[]  SumI3OutMin=[]  SumI3OutMax=[]  SumI4OutMin=[]  SumI4OutMax=[]  SumDOutMin=[]  SumDOutMax=[]  DifferentiatorOutMin=[]  DifferentiatorOutMax=[]  FilterDiffOutCoefMin=[]  FilterDiffOutCoefMax=[]  ReciprocalOutMin=[]  ReciprocalOutMax=[]  SumDenOutMin=[]  SumDenOutMax=[]  SumNumOutMin=[]  SumNumOutMax=[]  DivideOutMin=[]  DivideOutMax=[]  UdiffTsProdOutMin=[]  UdiffTsProdOutMax=[]  NTsProdOutMin=[]  NTsProdOutMax=[]  UintegralTsProdOutMin=[]  UintegralTsProdOutMax=[]  UngainTsProdOutMin=[]  UngainTsProdOutMax=[]  ClampingZeroOutDataTypeStr=Inherit: Inherit via back propagation  ClampingZeroOutMin=[]  ClampingZeroOutMax=[]  FilterDenConstantOutDataTypeStr=Inherit: Inherit via back propagation  FilterDenConstantOutMin=[]  FilterDenConstantOutMax=[]  PCopyOutDataTypeStr=Inherit: Inherit via back propagation  PCopyOutMin=[]  PCopyOutMax=[]  NCopyOutDataTypeStr=Inherit: Inherit via back propagation  NCopyOutMin=[]  NCopyOutMax=[]  IntegratorContinuousStateAttributes=''  IntegratorStateMustResolveToSignalObject=off  IntegratorRTWStateStorageClass=Auto  FilterContinuousStateAttributes=''  FilterStateMustResolveToSignalObject=off  FilterRTWStateStorageClass=Auto  ParallelPVariant=InternalParameters  IdealPVariant=Disabled  IVariant=InternalParameters  DVariant=InternalParameters  IntegratorVariant=Continuous  SatVariant=Disabled  AWVariant=Passthrough  PCopyVariant=Disabled  TRVariant=Disabled  FdbkBlocksVariant=Forward  IdealPFdbkVariant=Disabled  SatFdbkVariant=Disabled  DerivativeFilterVariant=ContFilter  NVariant=InternalParameters  NCopyVariant=Disabled  FilterICVariant=InternalICsFilter  IntegratorICVariant=InternalICs  ExternalResetVariant=Disabled  TRSumVariant=Passthrough  SumFdbkVariant=Disabled  SumVariant=Sum_PID  TsampFilterVariant=InternalTs  TsampNgainVariant=Passthrough  TsampIntegralVariant=Disabled_SignalSpec  ExternalSaturationOutDataTypeStr=Inherit: Same as second input
  Product : Product
  Saturation 6V1 : Saturate  UpperLimit=5  LowerLimit=-5
  Saturation 6V2 : Saturate  UpperLimit=5  LowerLimit=-5
  Saturation 6V3 : Saturate  UpperLimit=5  LowerLimit=-5
  Scope : Scope
  Scope1 : Scope
  Scope2 : Scope
  Step : Step  Time=0  After=-1  SampleTime=0
  magTorqueMatrix : Outport
  momentoDipolar : Outport  Port=2
  wires:
  Corrección Y/1(H_error) -> PID Controller1/1
  Corrección X/1(H_error) -> PID Controller3/1
  Step/1 -> Product/2
  Geomagetic/1 -> Product/1
  Cross Product2/1 -> Add/3  "MgtZ"
  Mgt_ejeZ/1 -> Cross Product2/1
  Momento Dipolar Z/1 -> Mgt_ejeZ/1
  Saturation 6V3/1 -> Momento Dipolar Z/1  "PWR_mgt Y"
  PID Controller2/1 -> Manual Switch2/1
  Manual Switch2/1 -> Saturation 6V3/1
  MATLAB Function/2(momentoDipolar) -> Contribucion de cada Mgt2/2
  Add1/1 -> momentoDipolar/1, Contribucion de cada Mgt2/1
  MATLAB Function/1(magTorqueMatrix) -> Contribucion de cada Mgt1/2
  Add/1 -> magTorqueMatrix/1, Scope/1, Contribucion de cada Mgt1/1
  Cross Product1/1 -> Add/2, Contribucion de cada Mgt/2  "MgtY"
  Mgt_ejeY/1 -> Cross Product1/1
  Momento Dipolar Y/1 -> Mgt_ejeY/1, Add1/2
  Saturation 6V2/1 -> Momento Dipolar Y/1, MATLAB Function/3(voltageY), Scope2/1  "PWR_mgt Y"
  Cross Product/1 -> Contribucion de cada Mgt/1, Add/1  "MgtX"
  Mgt_ejeX/1 -> Cross Product/1
  Momento Dipolar X/1 -> Mgt_ejeX/1, Add1/1
  Manual Switch1/1 -> Saturation 6V1/1
  Constant1/1 -> Manual Switch1/1
  Constant/1 -> Manual Switch/2, MATLAB Function/4(voltageZ), Manual Switch2/2
  PID Controller1/1 -> Manual Switch/1
  Manual Switch/1 -> Saturation 6V2/1
  Product/1 -> Cross Product/2, Cross Product1/2, Cross Product2/2, MATLAB Function/1(B), Corrección X/2(B), Corrección Y/2(B)
  Hz_error/1 -> Corrección X/1("H_error "), Corrección Y/1("H_error "), PID Controller2/1
  Saturation 6V1/1 -> Momento Dipolar X/1, MATLAB Function/2(voltageX), Scope1/1  "PWR_mgt X"
  PID Controller3/1 -> Manual Switch1/2

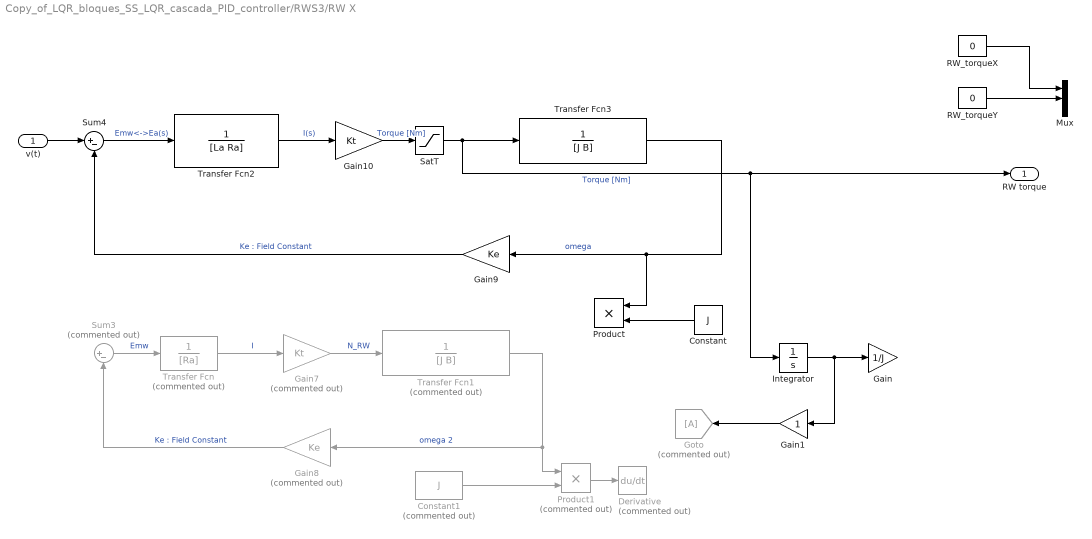
== system Copy_of_LQR_bloques_SS_LQR_cascada_PID_controller/RWS3/RW X ==
  v(t) : Inport
  Constant : Constant  Value=J
  Constant1 : Constant  Commented=on  Value=J
  Derivative : Derivative  Commented=on
  Gain : Gain  Gain=1/J
  Gain1 : Gain
  Gain10 : Gain  Gain=Kt
  Gain7 : Gain  Commented=on  Gain=Kt
  Gain8 : Gain  Commented=on  Gain=Ke
  Gain9 : Gain  Gain=Ke
  Goto : Goto  Commented=on
  Integrator : Integrator
  Mux : Mux  Inputs=3
  Product : Product
  Product1 : Product  Commented=on
  RW_torqueX : Constant  Value=0
  RW_torqueY : Constant  Value=0
  SatT : Saturate  UpperLimit=T_max  LowerLimit=-T_max
  Sum3 : Sum  Commented=on  Inputs=|+-
  Sum4 : Sum  Inputs=|+-
  Transfer Fcn : TransferFcn  Commented=on  Denominator=[Ra]
  Transfer Fcn1 : TransferFcn  Commented=on  Denominator=[J B]
  Transfer Fcn2 : TransferFcn  Denominator=[La Ra]
  Transfer Fcn3 : TransferFcn  Denominator=[J B]
  RW torque : Outport  VectorParamsAs1DForOutWhenUnconnected=off
  wires:
  SatT/1 -> Transfer Fcn3/1, Integrator/1, RW torque/1  "Torque [Nm]"
  Gain1/1 -> Goto/1
  Gain10/1 -> SatT/1  "Torque [Nm]"
  RW_torqueY/1 -> Mux/2
  RW_torqueX/1 -> Mux/1
  Gain8/1 -> Sum3/2  "Ke : Field Constant"
  Transfer Fcn/1 -> Gain7/1  "I"
  Sum3/1 -> Transfer Fcn/1  "Emw"
  Gain7/1 -> Transfer Fcn1/1  "N_RW"
  Transfer Fcn1/1 -> Gain8/1, Product1/1  "omega 2"
  Constant1/1 -> Product1/2
  Product1/1 -> Derivative/1
  v(t)/1 -> Sum4/1
  Integrator/1 -> Gain/1, Gain1/1
  Constant/1 -> Product/2
  Transfer Fcn3/1 -> Product/1, Gain9/1  "omega"
  Gain9/1 -> Sum4/2  "Ke : Field Constant"
  Sum4/1 -> Transfer Fcn2/1  "Emw<->Ea(s)"
  Transfer Fcn2/1 -> Gain10/1  "I(s)"

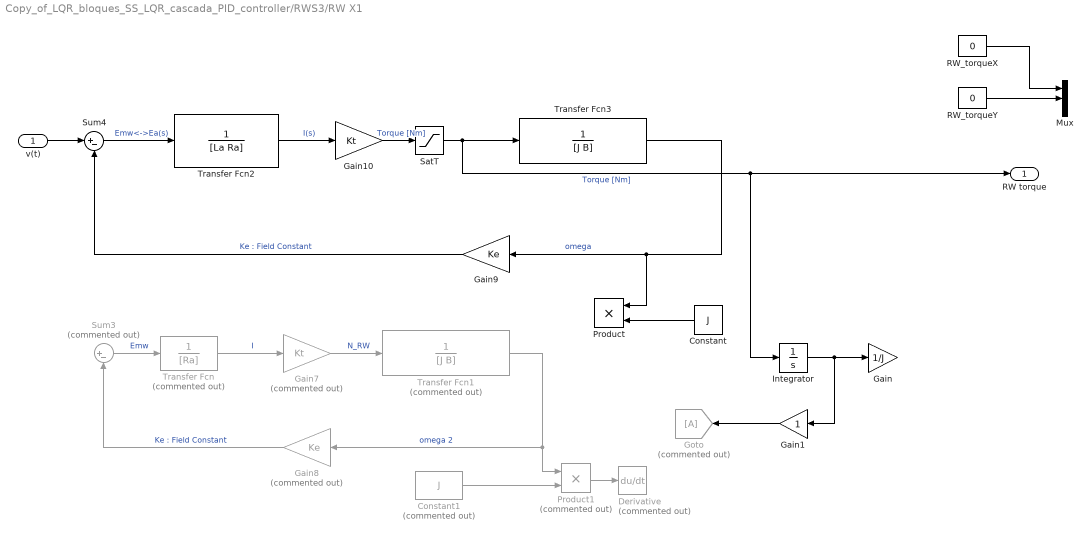
== system Copy_of_LQR_bloques_SS_LQR_cascada_PID_controller/RWS3/RW X1 ==
  v(t) : Inport
  Constant : Constant  Value=J
  Constant1 : Constant  Commented=on  Value=J
  Derivative : Derivative  Commented=on
  Gain : Gain  Gain=1/J
  Gain1 : Gain
  Gain10 : Gain  Gain=Kt
  Gain7 : Gain  Commented=on  Gain=Kt
  Gain8 : Gain  Commented=on  Gain=Ke
  Gain9 : Gain  Gain=Ke
  Goto : Goto  Commented=on
  Integrator : Integrator
  Mux : Mux  Inputs=3
  Product : Product
  Product1 : Product  Commented=on
  RW_torqueX : Constant  Value=0
  RW_torqueY : Constant  Value=0
  SatT : Saturate  UpperLimit=T_max  LowerLimit=-T_max
  Sum3 : Sum  Commented=on  Inputs=|+-
  Sum4 : Sum  Inputs=|+-
  Transfer Fcn : TransferFcn  Commented=on  Denominator=[Ra]
  Transfer Fcn1 : TransferFcn  Commented=on  Denominator=[J B]
  Transfer Fcn2 : TransferFcn  Denominator=[La Ra]
  Transfer Fcn3 : TransferFcn  Denominator=[J B]
  RW torque : Outport  VectorParamsAs1DForOutWhenUnconnected=off
  wires:
  Transfer Fcn2/1 -> Gain10/1  "I(s)"
  Sum4/1 -> Transfer Fcn2/1  "Emw<->Ea(s)"
  Gain9/1 -> Sum4/2  "Ke : Field Constant"
  Transfer Fcn3/1 -> Gain9/1, Product/1  "omega"
  Constant/1 -> Product/2
  Integrator/1 -> Gain1/1, Gain/1
  v(t)/1 -> Sum4/1
  Product1/1 -> Derivative/1
  Constant1/1 -> Product1/2
  Transfer Fcn1/1 -> Product1/1, Gain8/1  "omega 2"
  Gain7/1 -> Transfer Fcn1/1  "N_RW"
  Sum3/1 -> Transfer Fcn/1  "Emw"
  Transfer Fcn/1 -> Gain7/1  "I"
  Gain8/1 -> Sum3/2  "Ke : Field Constant"
  RW_torqueX/1 -> Mux/1
  RW_torqueY/1 -> Mux/2
  Gain10/1 -> SatT/1  "Torque [Nm]"
  Gain1/1 -> Goto/1
  SatT/1 -> RW torque/1, Integrator/1, Transfer Fcn3/1  "Torque [Nm]"

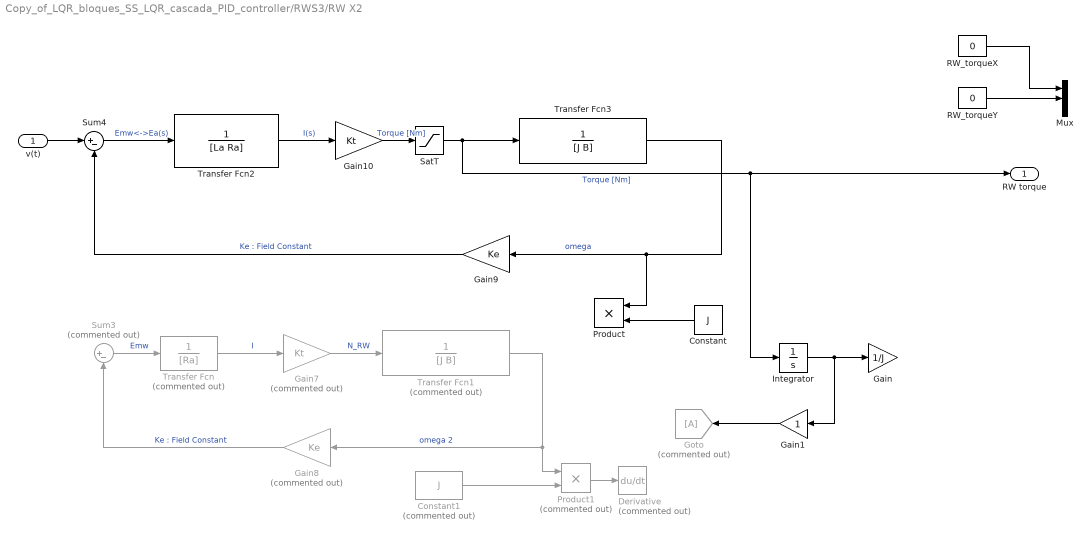
== system Copy_of_LQR_bloques_SS_LQR_cascada_PID_controller/RWS3/RW X2 ==
  v(t) : Inport
  Constant : Constant  Value=J
  Constant1 : Constant  Commented=on  Value=J
  Derivative : Derivative  Commented=on
  Gain : Gain  Gain=1/J
  Gain1 : Gain
  Gain10 : Gain  Gain=Kt
  Gain7 : Gain  Commented=on  Gain=Kt
  Gain8 : Gain  Commented=on  Gain=Ke
  Gain9 : Gain  Gain=Ke
  Goto : Goto  Commented=on
  Integrator : Integrator
  Mux : Mux  Inputs=3
  Product : Product
  Product1 : Product  Commented=on
  RW_torqueX : Constant  Value=0
  RW_torqueY : Constant  Value=0
  SatT : Saturate  UpperLimit=T_max  LowerLimit=-T_max
  Sum3 : Sum  Commented=on  Inputs=|+-
  Sum4 : Sum  Inputs=|+-
  Transfer Fcn : TransferFcn  Commented=on  Denominator=[Ra]
  Transfer Fcn1 : TransferFcn  Commented=on  Denominator=[J B]
  Transfer Fcn2 : TransferFcn  Denominator=[La Ra]
  Transfer Fcn3 : TransferFcn  Denominator=[J B]
  RW torque : Outport  VectorParamsAs1DForOutWhenUnconnected=off
  wires:
  SatT/1 -> Transfer Fcn3/1, Integrator/1, RW torque/1  "Torque [Nm]"
  Gain1/1 -> Goto/1
  Gain10/1 -> SatT/1  "Torque [Nm]"
  RW_torqueY/1 -> Mux/2
  RW_torqueX/1 -> Mux/1
  Gain8/1 -> Sum3/2  "Ke : Field Constant"
  Transfer Fcn/1 -> Gain7/1  "I"
  Sum3/1 -> Transfer Fcn/1  "Emw"
  Gain7/1 -> Transfer Fcn1/1  "N_RW"
  Transfer Fcn1/1 -> Gain8/1, Product1/1  "omega 2"
  Constant1/1 -> Product1/2
  Product1/1 -> Derivative/1
  v(t)/1 -> Sum4/1
  Integrator/1 -> Gain/1, Gain1/1
  Constant/1 -> Product/2
  Transfer Fcn3/1 -> Product/1, Gain9/1  "omega"
  Gain9/1 -> Sum4/2  "Ke : Field Constant"
  Sum4/1 -> Transfer Fcn2/1  "Emw<->Ea(s)"
  Transfer Fcn2/1 -> Gain10/1  "I(s)"

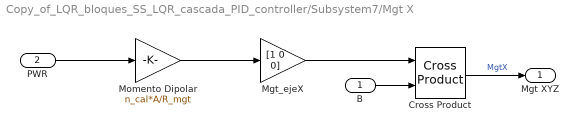
== system Copy_of_LQR_bloques_SS_LQR_cascada_PID_controller/Subsystem7/Mgt X ==
  B : Inport
  PWR : Inport  Port=2
  Cross Product : matrix_library/Cross Product
  Mgt_ejeX : Gain  Gain=[1 0 0]
  "Momento Dipolar " : Gain  Gain=n_cal*A/R_mgt
  Mgt XYZ : Outport
  wires:
  "Momento Dipolar "/1 -> Mgt_ejeX/1
  Mgt_ejeX/1 -> Cross Product/1
  Cross Product/1 -> Mgt XYZ/1  "MgtX"
  PWR/1 -> "Momento Dipolar "/1
  B/1 -> Cross Product/2

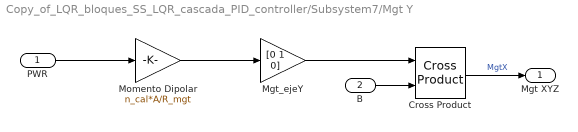
== system Copy_of_LQR_bloques_SS_LQR_cascada_PID_controller/Subsystem7/Mgt Y ==
  PWR : Inport
  B : Inport  Port=2
  Cross Product : matrix_library/Cross Product
  Mgt_ejeY : Gain  Gain=[0 1 0]
  "Momento Dipolar " : Gain  Gain=n_cal*A/R_mgt
  Mgt XYZ : Outport
  wires:
  B/1 -> Cross Product/2
  PWR/1 -> "Momento Dipolar "/1
  Cross Product/1 -> Mgt XYZ/1  "MgtX"
  Mgt_ejeY/1 -> Cross Product/1
  "Momento Dipolar "/1 -> Mgt_ejeY/1

== matlab function Copy_of_LQR_bloques_SS_LQR_cascada_PID_controller/Subsystem7/Corrección X ==
  data: T_error input; B input; T_error output
function T_error = fcn(T_error,B)

if (B(2)> 0)
    HGain =1;
else
    HGain =- 1;

end
T_error = T_error*HGain; 
end

== matlab function Copy_of_LQR_bloques_SS_LQR_cascada_PID_controller/Subsystem7/Corrección Y ==
  data: T_error input; B input; T_error output
function T_error = MgtY_correction(T_error,B)
HGain =1;

if (B(1)>= 0)
    HGain =-1;
else
    HGain =1 ;

end
T_error = T_error*HGain; 
end

== matlab function Copy_of_LQR_bloques_SS_LQR_cascada_PID_controller/Subsystem8/Extract B ==
  data: B_cal input; XYZ_Magnetic output size=[3,1]; time input
function XYZ_Magnetic = fcn(B_cal,time)

index= 1+round(time);
s = size(B_cal);
if index> s(2)
    XYZ_Magnetic = B_cal(:,s(2));
else
    XYZ_Magnetic = B_cal(:,index);
end

== matlab function Copy_of_LQR_bloques_SS_LQR_cascada_PID_controller/Subsystem8/MATLAB Function ==
  data: NEDMagnetic input; RPY_Magnetic output; RPY input
function RPY_Magnetic = RPY_Magnetic(NEDMagnetic,RPY)

R = RPY(1);
P= RPY(2);
Y = RPY(3);



C_NED2ENU = [0 1 0;
             1 0 0
             0 0 -1];
C_RPY2ENU = [sin(Y)*cos(P) cos(R)*cos(Y)+sin(R)*sin(Y)*sin(P) -sin(R)*cos(Y)+cos(R)*sin(Y)*sin(P);
    cos(Y)*cos(P) -cos(R)*sin(Y)+sin(R)*cos(Y)*sin(P) sin(R)*sin(Y)+cos(R)*cos(Y)*sin(P);
    sin(P) -sin(R)*cos(P) -cos(R)*cos(P)];

C_ENU2RPY = C_RPY2ENU^-1; 

RPY_Magnetic = C_ENU2RPY*C_NED2ENU*NEDMagnetic; 


end

== matlab function Copy_of_LQR_bloques_SS_LQR_cascada_PID_controller/Subsystem9/Corrección X ==
  data: H_error input; B input; H_error output
function H_error = fcn(H_error,B)

if (B(2)> 0)
    HGain =1;
else
    HGain =- 1;

end
H_error = H_error*HGain; 
end

== matlab function Copy_of_LQR_bloques_SS_LQR_cascada_PID_controller/Subsystem9/Corrección Y ==
  data: H_error input; B input; H_error output
function H_error = fcn(H_error,B)

if (B(1)> 0)
    HGain =-1;
else
    HGain =1 ;

end
H_error = H_error*HGain; 
end

== matlab function Copy_of_LQR_bloques_SS_LQR_cascada_PID_controller/Subsystem9/MATLAB Function ==
  data: B input; magTorqueMatrix output; voltageX input; voltageY input; voltageZ input; momentoDipolar output
function [magTorqueMatrix,momentoDipolar] = magTorqueFunction(B,voltageX,voltageY,voltageZ)

%d = 1.45e-2; % Diametro mgt [m]
d = 1.45e-2; % Diametro mgt [m]
A =d^2*pi/4;

%n=sqrt(L*l/(mu_0*mu_r*A)); % # Vueltas 
n = 5412;

%R = 50.7 ;% Resistencia mgt [Ohm];
R = 30 ;% Resistencia mgt [Ohm];
ix = voltageX/R;
iy = voltageY/R;
iz = voltageZ/R;

% M = [n*ix*A n*iy*A n*iz*A]';
% 
% magTorqueMatrix = -skew(B)*M;

magTorqueMatrix_X = cross(n*ix*A*[1 0 0],B);
magTorqueMatrix_Y = cross(n*iy*A*[0 1 0],B);
magTorqueMatrix_Z = cross(n*iz*A*[0 0 1],B);
 momentoDipolar = [n*ix*A n*iy*A n*iz*A];

magTorqueMatrix = magTorqueMatrix_X+magTorqueMatrix_Y+magTorqueMatrix_Z;
